simulink model "model"  (R2022a)
settings: Solver=ode4  StartTime=0.0  StopTime=Inf  FixedStep=5e-3  RelTol=1e-3
values from neighbouring files (symbols this model uses):
  emin = 0.05    [simulate.m]
  poseR0 = [2,2,pi/4]    [simulate.m]
  xg = 0    [simulate.m]
  yg = 0    [simulate.m]
libraries: simulink x1
settings Model: PacingRate=0.800000  Creator=mateu  LastModifiedBy=mateu

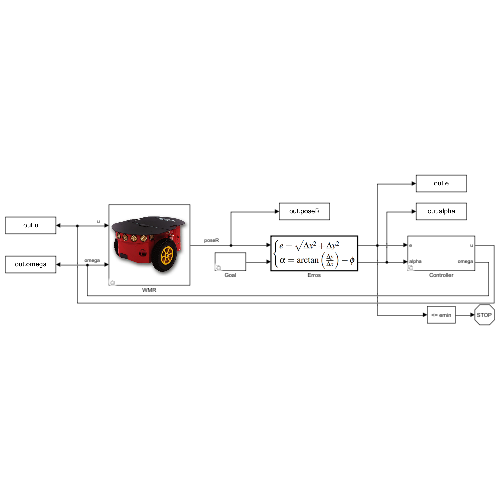
[thumbnail: Simulink's stored preview of the top-level diagram]
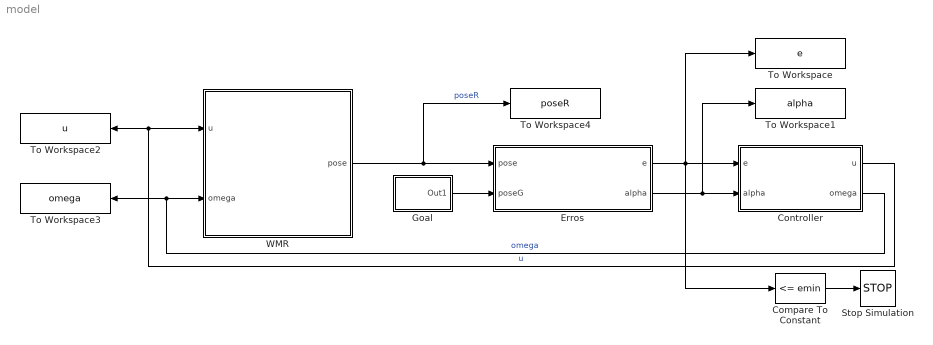
== system model ==
  Compare To Constant : simulink/Logic and Bit Operations/Compare To Constant  relop=<=  const=emin  OutDataTypeStr=boolean
  Controller : Subsystem  Variant=on
      mask Display: image('$imagefile'); % Use "Edit Image" on toolstrip to change.
  Erros : MATLAB Function  TreatAsAtomicUnit=on
  Goal : Subsystem  Variant=on
      mask Display: image('$imagefile'); % Use "Edit Image" on toolstrip to change.
  Stop Simulation : Stop
  To Workspace : ToWorkspace  VariableName=e  SaveFormat=Timeseries  SampleTime=-1
  To Workspace1 : ToWorkspace  VariableName=alpha  SaveFormat=Timeseries  SampleTime=-1
  To Workspace2 : ToWorkspace  VariableName=u  SaveFormat=Timeseries  SampleTime=-1
  To Workspace3 : ToWorkspace  VariableName=omega  SaveFormat=Timeseries  SampleTime=-1
  To Workspace4 : ToWorkspace  VariableName=poseR  SaveFormat=Timeseries  SampleTime=-1
  WMR : Subsystem  Variant=on
      mask Display: image('$imagefile'); % Use "Edit Image" on toolstrip to change.
  wires:
  WMR/1(pose) -> To Workspace4/1, Erros/1(pose)  "poseR"
  Erros/1(e) -> To Workspace/1, Controller/1(e), Compare To Constant/1
  Erros/2(alpha) -> Controller/2(alpha), To Workspace1/1
  Controller/2(omega) -> To Workspace3/1, WMR/2(omega)  "omega"
  Controller/1(u) -> To Workspace2/1, WMR/1(u)  "u"
  Goal/1(Out1) -> Erros/2(poseG)
  Compare To Constant/1 -> Stop Simulation/1

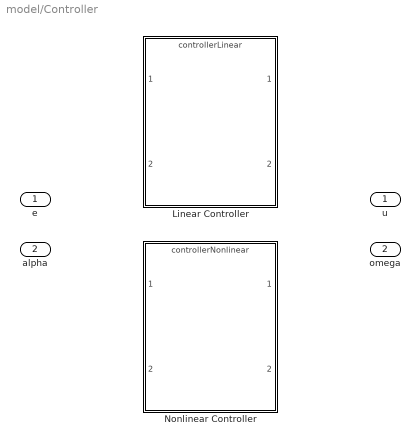
== system model/Controller ==
  e : Inport
  alpha : Inport  Port=2
  Linear Controller : ModelReference  DisableCoverage=on  ModelNameDialog=controllerLinear  VariantControl=CONTROL_LINEAR  ModelReferenceVersion=1.3
  Nonlinear Controller : ModelReference  ModelNameDialog=controllerNonlinear  VariantControl=CONTROL_NONLINEAR  ModelReferenceVersion=1.4
  u : Outport
  omega : Outport  Port=2

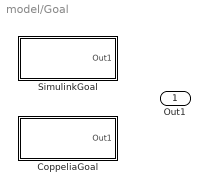
== system model/Goal ==
  CoppeliaGoal : Subsystem  VariantControl=GOAL_COPPELIA
  SimulinkGoal : Subsystem  VariantControl=GOAL_SIMULINK
  Out1 : Outport

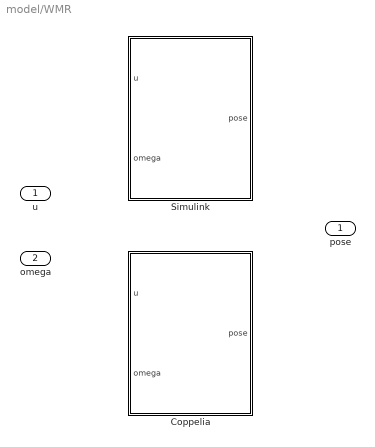
== system model/WMR ==
  u : Inport
  omega : Inport  Port=2
  Coppelia : Subsystem  VariantControl=UNICYCLE_COPPELIA
  Simulink : Subsystem  VariantControl=UNICYCLE_SIMULINK
  pose : Outport

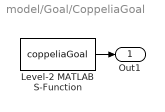
== system model/Goal/CoppeliaGoal ==
  Level-2 MATLAB S-Function : M-S-Function  FunctionName=coppeliaGoal
  Out1 : Outport
  wires:
  Level-2 MATLAB S-Function/1 -> Out1/1

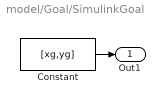
== system model/Goal/SimulinkGoal ==
  Constant : Constant  Value=[xg,yg]
  Out1 : Outport
  wires:
  Constant/1 -> Out1/1

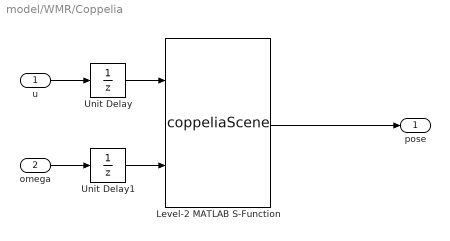
== system model/WMR/Coppelia ==
  u : Inport
  omega : Inport  Port=2
  Level-2 MATLAB S-Function : M-S-Function  FunctionName=coppeliaScene  Parameters=poseR0
  Unit Delay : UnitDelay  SampleTime=-1  HasFrameUpgradeWarning=on
  Unit Delay1 : UnitDelay  SampleTime=-1  HasFrameUpgradeWarning=on
  pose : Outport
  wires:
  u/1 -> Unit Delay/1
  omega/1 -> Unit Delay1/1
  Level-2 MATLAB S-Function/1 -> pose/1
  Unit Delay/1 -> Level-2 MATLAB S-Function/1
  Unit Delay1/1 -> Level-2 MATLAB S-Function/2

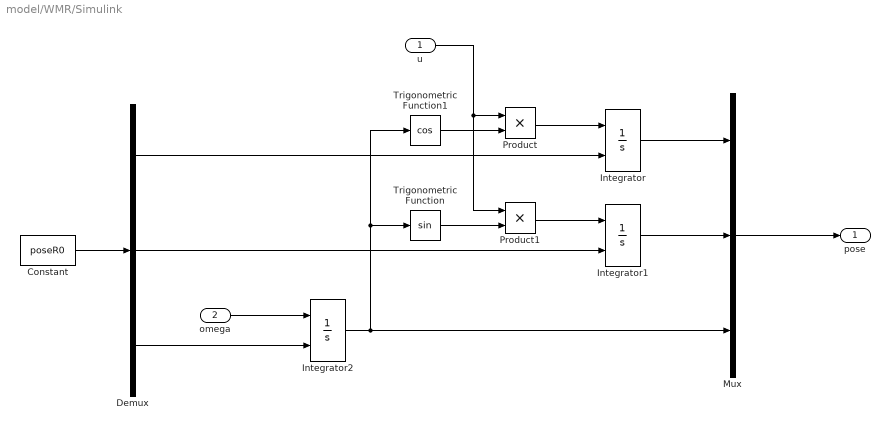
== system model/WMR/Simulink ==
  u : Inport
  omega : Inport  Port=2
  Constant : Constant  Value=poseR0
  Demux : Demux  Outputs=3
  Integrator : Integrator  InitialConditionSource=external
  Integrator1 : Integrator  InitialConditionSource=external
  Integrator2 : Integrator  InitialConditionSource=external
  Mux : Mux  Inputs=3
  Product : Product
  Product1 : Product
  Trigonometric Function : Trigonometry
  Trigonometric Function1 : Trigonometry  Operator=cos
  pose : Outport
  wires:
  Demux/3 -> Integrator2/2
  Constant/1 -> Demux/1
  Mux/1 -> pose/1
  Integrator2/1 -> Trigonometric Function1/1, Trigonometric Function/1, Mux/3
  Demux/1 -> Integrator/2
  omega/1 -> Integrator2/1
  Product1/1 -> Integrator1/1
  Product/1 -> Integrator/1
  Trigonometric Function1/1 -> Product/2
  Trigonometric Function/1 -> Product1/2
  Demux/2 -> Integrator1/2
  u/1 -> Product/1, Product1/1
  Integrator1/1 -> Mux/2
  Integrator/1 -> Mux/1

== matlab function model/Erros ==
  settings: updateMethod=DISCRETE  sampleTime=0.05
  data: pose input; e output; poseG input; alpha output
function [e,alpha] = errors(pose,poseG)

deltaX = poseG(1)-pose(1); deltaY = poseG(2)-pose(2);
phi = pose(3);

e = sqrt(deltaX^2 + deltaY^2);
alpha = atan2(deltaY,deltaX) - phi;
